simulink model "ECGModel"  (R2022a)
settings: Solver=VariableStepAuto  StartTime=0.0  StopTime=10.0  RelTol=1e-3
settings Model: Creator=User  LastModifiedBy=User

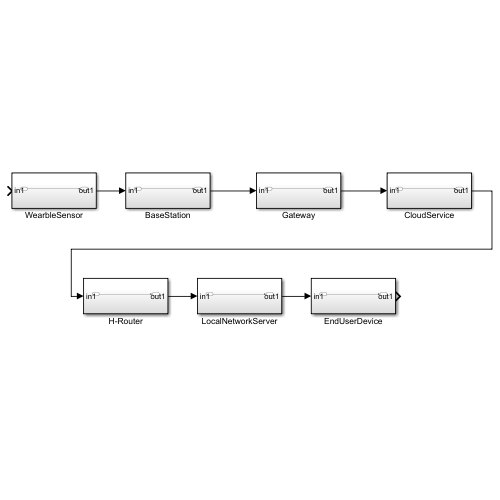
[thumbnail: Simulink's stored preview of the top-level diagram]
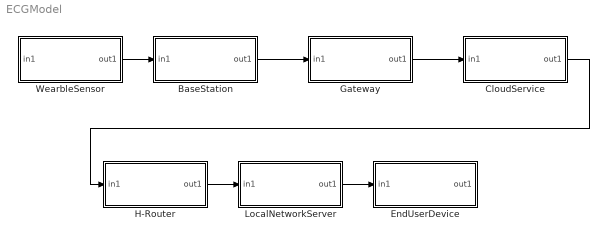
== system ECGModel ==
  BaseStation : Subsystem
  CloudService : Subsystem
  EndUserDevice : Subsystem
  Gateway : Subsystem
  H-Router : Subsystem
  LocalNetworkServer : Subsystem
  WearbleSensor : Subsystem
  wires:
  WearbleSensor/1(out1) -> BaseStation/1(in1)
  BaseStation/1(out1) -> Gateway/1(in1)
  Gateway/1(out1) -> CloudService/1(in1)
  CloudService/1(out1) -> H-Router/1(in1)
  H-Router/1(out1) -> LocalNetworkServer/1(in1)
  LocalNetworkServer/1(out1) -> EndUserDevice/1(in1)

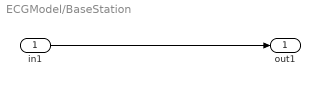
== system ECGModel/BaseStation ==
  in1 : Inport
  out1 : Outport
  wires:
  in1/1 -> out1/1

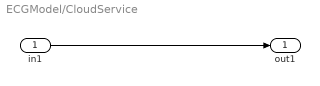
== system ECGModel/CloudService ==
  in1 : Inport
  out1 : Outport
  wires:
  in1/1 -> out1/1

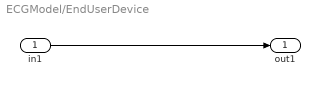
== system ECGModel/EndUserDevice ==
  in1 : Inport
  out1 : Outport
  wires:
  in1/1 -> out1/1

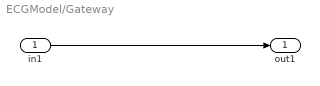
== system ECGModel/Gateway ==
  in1 : Inport
  out1 : Outport
  wires:
  in1/1 -> out1/1

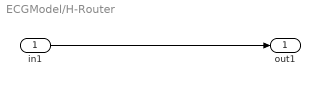
== system ECGModel/H-Router ==
  in1 : Inport
  out1 : Outport
  wires:
  in1/1 -> out1/1

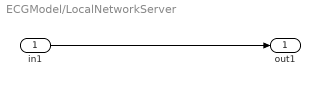
== system ECGModel/LocalNetworkServer ==
  in1 : Inport
  out1 : Outport
  wires:
  in1/1 -> out1/1

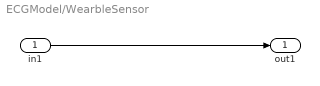
== system ECGModel/WearbleSensor ==
  in1 : Inport
  out1 : Outport
  wires:
  in1/1 -> out1/1
